simulink model "SVFB_LocalObserver"  (R2024a)
settings: Solver=VariableStepAuto  StartTime=0.0  StopTime=Tf  RelTol=1e-3
values from neighbouring files (symbols this model uses):
  A = [0 1; 880.87 0]    [main.m]
  B = [0; -9.9453]    [main.m]
  C = [708.27 0]    [main.m]
  K0 = place(A, B, p_desired_tracking)    [main.m]
  L_luemb = place(A', C', desired_poles)'    [main.m]
  S0_x0 = [10 0]'    [main.m]
undefined symbols (not defined in the file or in its folder): err
settings Model: Creator=aless  LastModifiedBy=Stefano

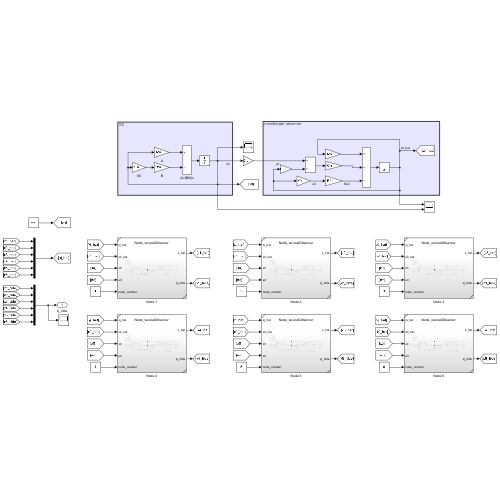
[thumbnail: Simulink's stored preview of the top-level diagram]
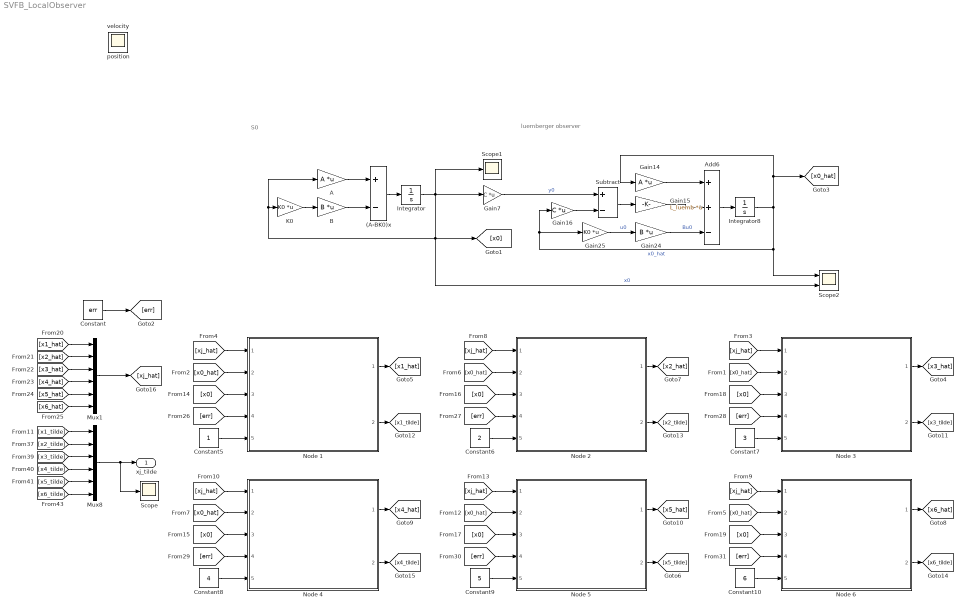
== system SVFB_LocalObserver ==
  note: luemberger observer
  note: S0
  (A-BK0)x : Sum  Inputs=+-
  A : Gain  Gain=A  Multiplication=Matrix(K*u)
  Add6 : Sum  Inputs=++-
  B : Gain  Gain=B  Multiplication=Matrix(K*u)
  Constant : Constant  Value=err
  Constant10 : Constant  Value=6
  Constant5 : Constant
  Constant6 : Constant  Value=2
  Constant7 : Constant  Value=3
  Constant8 : Constant  Value=4
  Constant9 : Constant  Value=5
  Gain14 : Gain  Gain=A  Multiplication=Matrix(K*u)
  Gain15 : Gain  Gain=L_luemb  Multiplication=Matrix(K*u)
  Gain16 : Gain  Gain=C  Multiplication=Matrix(K*u)
  Gain24 : Gain  Gain=B  Multiplication=Matrix(K*u)
  Gain25 : Gain  Gain=K0  Multiplication=Matrix(K*u)
  Gain7 : Gain  Gain=C  Multiplication=Matrix(K*u)
  Integrator : Integrator  InitialCondition=S0_x0
  Integrator8 : Integrator  InitialCondition=S0_x0
  K0 : Gain  Gain=K0  Multiplication=Matrix(K*u)
  Mux1 : Mux  Inputs=6
  Mux8 : Mux  Inputs=6
  Node {1..6} (6 alike) : Subsystem  ReferencedSubsystem=Node_wLocalObserver
  Scope : Scope
  Scope1 : Scope
  Scope2 : Scope  NumInputPorts=2
  Subtract : Sum  Inputs=+-
  xj_tilde : Outport
  position : Scope
  velocity : Scope
  wires:
  A/1 -> (A-BK0)x/1
  Integrator8/1 -> Gain14/1, [x0_hat], Scope2/1, Gain25/1, Gain16/1  "x0_hat"
  Add6/1 -> Integrator8/1
  Gain7/1 -> Subtract/1  "y0"
  B/1 -> (A-BK0)x/2
  Gain15/1 -> Add6/2
  Subtract/1 -> Gain15/1
  (A-BK0)x/1 -> Integrator/1
  Integrator/1 -> Scope2/2, [x0], A/1, K0/1, Gain7/1, Scope1/1  "x0"
  Gain14/1 -> Add6/1
  Gain16/1 -> Subtract/2
  [x5_tilde] -> Mux8/5
  [x3_tilde] -> Mux8/3
  [x2_tilde] -> Mux8/2
  [x6_tilde] -> Mux8/6
  [x1_tilde] -> Mux8/1
  [x4_tilde] -> Mux8/4
  K0/1 -> B/1
  [x0_hat] -> Node 1/2
  [xj_hat] -> Node 1/1
  Constant5/1 -> Node 1/5
  Node 1/1 -> [x1_hat]
  Constant6/1 -> Node 2/5
  [xj_hat] -> Node 2/1
  [x0_hat] -> Node 2/2
  Node 2/1 -> [x2_hat]
  Node 3/1 -> [x3_hat]
  [x0_hat] -> Node 3/2
  [xj_hat] -> Node 3/1
  Constant7/1 -> Node 3/5
  [xj_hat] -> Node 6/1
  [x0_hat] -> Node 6/2
  Node 6/1 -> [x6_hat]
  Node 5/1 -> [x5_hat]
  [x0_hat] -> Node 5/2
  [xj_hat] -> Node 5/1
  Node 4/1 -> [x4_hat]
  [xj_hat] -> Node 4/1
  [x0_hat] -> Node 4/2
  Mux8/1 -> Scope/1, xj_tilde/1
  Node 4/2 -> [x4_tilde]
  Node 1/2 -> [x1_tilde]
  Node 5/2 -> [x5_tilde]
  Node 6/2 -> [x6_tilde]
  Node 3/2 -> [x3_tilde]
  [x0] -> Node 1/3
  [x0] -> Node 4/3
  [x0] -> Node 3/3
  [x0] -> Node 6/3
  [x0] -> Node 5/3
  [x0] -> Node 2/3
  [x6_hat] -> Mux1/6
  [x2_hat] -> Mux1/2
  [x1_hat] -> Mux1/1
  Mux1/1 -> [xj_hat]
  [x3_hat] -> Mux1/3
  [x4_hat] -> Mux1/4
  [x5_hat] -> Mux1/5
  Gain25/1 -> Gain24/1  "u0"
  Gain24/1 -> Add6/3  "Bu0"
  [err] -> Node 1/4
  [err] -> Node 2/4
  [err] -> Node 3/4
  [err] -> Node 4/4
  Constant8/1 -> Node 4/5
  [err] -> Node 5/4
  Constant9/1 -> Node 5/5
  [err] -> Node 6/4
  Constant10/1 -> Node 6/5
  Constant/1 -> [err]
  Node 2/2 -> [x2_tilde]
